simulink model "four"  (R2023b)
settings: Solver=VariableStepAuto  StartTime=0.0  StopTime=10  RelTol=1e-3
undefined symbols (not defined in the file or in its folder): A, As, B_1, B_2, Bs, C_1, C_2, Cs, D_1, D_2, Ds, gamma1, K_1, K_2, L_1, Q_1, x_0
settings Model: Creator=evdokiiagalkina  LastModifiedBy=evdokiiagalkina

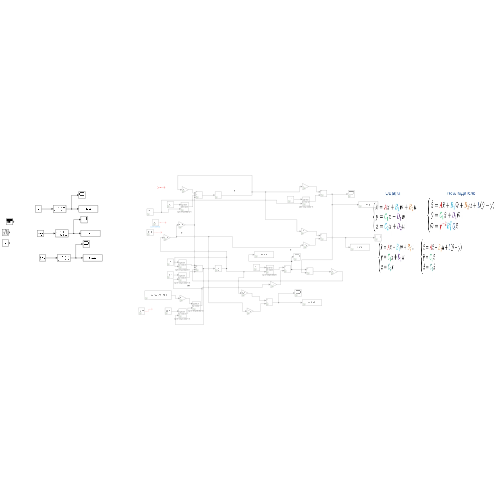
[thumbnail: Simulink's stored preview of the top-level diagram]
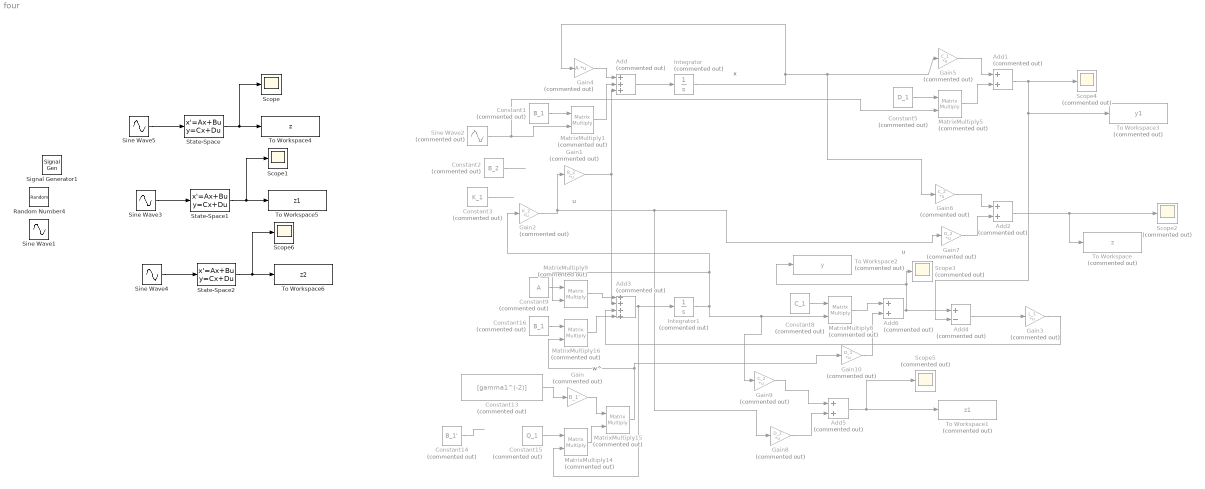
== system four ==
  note: w^
  note: x
  note: u
  note: u
  Add : Sum  Commented=on  Inputs=+++
  Add{1..2,5..6} (4 alike) : Sum  Commented=on
  Add3 : Sum  Commented=on  Inputs=++++
  Add4 : Sum  Commented=on  Inputs=+-
  Constant1 : Constant  Commented=on  Value=B_1
  Constant13 : Constant  Commented=on  Value=[gamma1^(-2)]
  Constant14 : Constant  Commented=on  Value=B_1'
  Constant15 : Constant  Commented=on  Value=Q_1
  Constant16 : Constant  Commented=on  Value=B_1
  Constant2 : Constant  Commented=on  Value=B_2
  Constant3 : Constant  Commented=on  Value=K_1
  Constant5 : Constant  Commented=on  Value=D_1
  Constant8 : Constant  Commented=on  Value=C_1
  Constant9 : Constant  Commented=on  Value=A
  Gain : Gain  Commented=on  Gain=B_1'
  Gain1 : Gain  Commented=on  Gain=B_2  Multiplication=Matrix(K*u)
  Gain10 : Gain  Commented=on  Gain=D_1  Multiplication=Matrix(K*u)
  Gain2 : Gain  Commented=on  Gain=K_2  Multiplication=Matrix(K*u)
  Gain3 : Gain  Commented=on  Gain=L_1  Multiplication=Matrix(K*u)
  Gain4 : Gain  Commented=on  Gain=A  Multiplication=Matrix(K*u)
  Gain5 : Gain  Commented=on  Gain=C_1  Multiplication=Matrix(K*u)
  Gain6 : Gain  Commented=on  Gain=C_2  Multiplication=Matrix(K*u)
  Gain7 : Gain  Commented=on  Gain=D_2  Multiplication=Matrix(K*u)
  Gain8 : Gain  Commented=on  Gain=D_2  Multiplication=Matrix(K*u)
  Gain9 : Gain  Commented=on  Gain=C_2  Multiplication=Matrix(K*u)
  Integrator : Integrator  Commented=on  InitialCondition=x_0
  Integrator1 : Integrator  Commented=on  InitialCondition=[4; 5]
  MatrixMultiply{1,5,8..9,14..16} (7 alike) : Product  Commented=on  Multiplication=Matrix(*)
  Random Number4 : RandomNumber  SampleTime=0.001
  Scope : Scope
  Scope1 : Scope
  Scope{2..5} (4 alike) : Scope  Commented=on
  Scope6 : Scope
  Signal Generator1 : SignalGenerator  WaveForm=square  Amplitude=0.1  Frequency=5  Units=rad/sec
  Sine Wave1 : Sin  SampleTime=0
  Sine Wave2 : Sin  Commented=on  Amplitude=5  SampleTime=0
  Sine Wave3 : Sin  Amplitude=10  Frequency=10  SampleTime=0
  Sine Wave4 : Sin  Amplitude=10  Frequency=30  SampleTime=0
  Sine Wave5 : Sin  Amplitude=10  SampleTime=0
  State-Space : StateSpace  A=As  B=Bs  C=Cs  D=Ds  InitialCondition=[1, 2; 3, 4]
  State-Space1 : StateSpace  A=As  B=Bs  C=Cs  D=Ds  InitialCondition=[1, 2; 3, 4]
  State-Space2 : StateSpace  A=As  B=Bs  C=Cs  D=Ds  InitialCondition=[1, 2; 3, 4]
  To Workspace : ToWorkspace  Commented=on  VariableName=z  SaveFormat=Timeseries  SampleTime=-1
  To Workspace1 : ToWorkspace  Commented=on  VariableName=z1  SaveFormat=Timeseries  SampleTime=-1
  To Workspace2 : ToWorkspace  Commented=on  VariableName=y  SaveFormat=Timeseries  SampleTime=-1
  To Workspace3 : ToWorkspace  Commented=on  VariableName=y1  SaveFormat=Timeseries  SampleTime=-1
  To Workspace4 : ToWorkspace  VariableName=z  SaveFormat=Timeseries  SampleTime=-1
  To Workspace5 : ToWorkspace  VariableName=z1  SaveFormat=Timeseries  SampleTime=-1
  To Workspace6 : ToWorkspace  VariableName=z2  SaveFormat=Timeseries  SampleTime=-1
  wires:
  MatrixMultiply1/1 -> Add/2
  Add5/1 -> Scope5/1, To Workspace1/1
  Sine Wave2/1 -> MatrixMultiply1/2, MatrixMultiply5/2
  MatrixMultiply9/1 -> Add3/1
  Gain4/1 -> Add/1
  Sine Wave5/1 -> State-Space/1
  ? -> ?
  Add3/1 -> MatrixMultiply14/2, Integrator1/1
  Constant1/1 -> MatrixMultiply1/1
  Integrator1/1 -> Gain2/1, MatrixMultiply9/2, Gain9/1, MatrixMultiply8/2
  Add4/1 -> Gain3/1
  Constant8/1 -> MatrixMultiply8/1
  Constant2/1 -> ?
  Add/1 -> Integrator/1
  MatrixMultiply8/1 -> Add6/1
  Gain7/1 -> Add2/2
  Gain6/1 -> Add2/1
  Gain2/1 -> Gain1/1, Gain8/1, Gain7/1
  Gain3/1 -> Add3/3
  Integrator/1 -> Gain4/1, Gain6/1, Gain5/1
  Constant9/1 -> MatrixMultiply9/1
  Add2/1 -> To Workspace/1, Scope2/1
  Gain5/1 -> Add1/1
  Add1/1 -> Scope4/1, To Workspace3/1, Add4/2
  Gain1/1 -> Add/3, Add3/2
  Constant3/1 -> ?
  MatrixMultiply5/1 -> Add1/2
  Constant5/1 -> MatrixMultiply5/1
  Gain8/1 -> Add5/2
  Gain9/1 -> Add5/1
  State-Space/1 -> To Workspace4/1, Scope/1
  Constant13/1 -> Gain/1
  Constant14/1 -> ?
  Constant15/1 -> MatrixMultiply14/1
  Gain/1 -> MatrixMultiply15/1
  MatrixMultiply14/1 -> MatrixMultiply15/2
  Constant16/1 -> MatrixMultiply16/1
  MatrixMultiply16/1 -> Add3/4
  Add6/1 -> Scope3/1, To Workspace2/1, Add4/1
  MatrixMultiply15/1 -> Gain10/1, MatrixMultiply16/2
  Gain10/1 -> Add6/2
  Sine Wave3/1 -> State-Space1/1
  State-Space1/1 -> To Workspace5/1, Scope1/1
  Sine Wave4/1 -> State-Space2/1
  State-Space2/1 -> To Workspace6/1, Scope6/1
